simulink library "can_control"  (R2023b)
settings: Solver=VariableStepAuto  StartTime=0.0  StopTime=10.0  RelTol=1e-3
undefined symbols (not defined in the file or in its folder): Data, Error, Extended, ID, Length, Remote, Timestamp
libraries: simulink x3, $bdroot x2, dspswit3 x1
settings Model: Creator=Olga  LastModifiedBy=Olga
settings SFSimCC: SimCustomHeaderCode="#include \"can_control.h\""  SimUserSources=.\can_control.c  SimAnalyzeCustomCode=on
settings RTWCC: RTWUseSimCustomCode=on  CustomHeaderCode="#include \"can_control.h\""  CustomSource=.\can_control.c

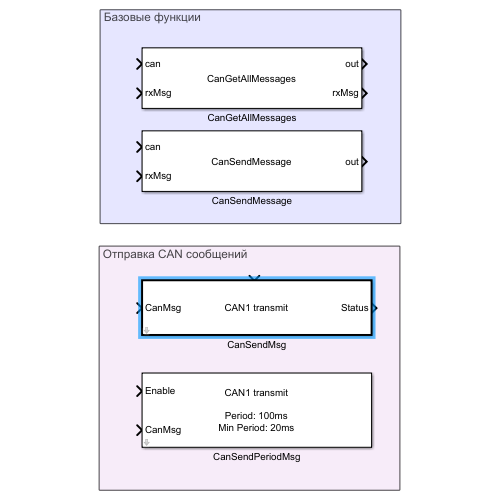
[thumbnail: Simulink's stored preview of the top-level diagram]
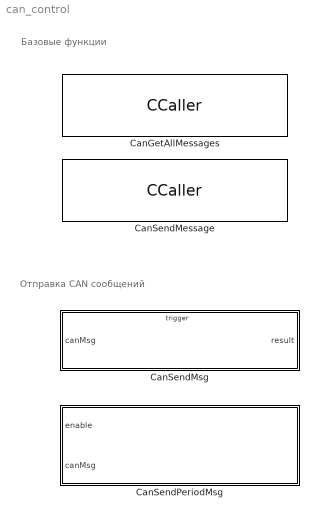
== system can_control ==
  note: Базовые функции
  note: Отправка CAN сообщений
  CanGetAllMessages : CCaller  FunctionName=CanGetAllMessages  PortSpecificationStruct="%)30     .    > 4   8    (     @         %    \"     ,    !     0         %  0 \"0    $    _    07)G3F%M90  4&]R=$YA;64 4V-O<&4     26YD97@     5'EP90      4VEZ90      27-';&]B86P   X    P    !@    @    $          4    (     0    ,    !         !   P!O=70 #@   #     &    \"     0         !0    @    !     P    $         $  # &]U=  .    .     8    (    !          %    \"     $    &     0         0    !@   $]U='!U=   #@   #@    &    \"     8         !0    @    !     0    $         \"0    @               X    X    !@    @    $          4    (     0    <    !         !     '    8F]O;&5A;@ .    ,     8    (    !          %    \"     $    !     0         0  $ ,0    X    P    !@    @    ) @        4    (     0    $    !          (  0      #@   #     &    \"     0         !0    @    !     P    $         $  # &-A;@ .    ,     8    (    !          %    \"     $    #     0         0  , 8V%N  X    X    !@    @    $          4    (     0    4    !         !     %    26YP=70    .    .     8    (    !@         %    \"     $    !     0         )    \"               #@   #@    &    \"     0         !0    @    !    !0    $         $     4   !I;G0S,@    X    P    !@    @    $          4    (     0    $    !         !   0 Q    #@   #     &    \"     D\"        !0    @    !     0    $          @ !       .    .     8    (    !          %    \"     $    %     0         0    !0   ')X37-G    #@   #@    &    \"     0         !0    @    !    !0    $         $     4   !R>$US9P    X   !     !@    @    $          4    (     0    L    !         !     +    26YP=71/=71P=70       X    X    !@    @    &          4    (     0    $    !          D    (            \\#\\.    0     8    (    !          %    \"     $    .     0         0    #@   $)U<SH@0T%.7TUS9U]T   .    ,     8    (    !          %    \"     $    \"     0         0  ( +3$   X    P    !@    @    ) @        4    (     0    $    !          (  0"
  CanSendMessage : CCaller  FunctionName=CanSendMessage  PortSpecificationStruct="%)30     .    < 4   8    (     @         %    \"     ,    !     0         %  0 \"0    $    _    07)G3F%M90  4&]R=$YA;64 4V-O<&4     26YD97@     5'EP90      4VEZ90      27-';&]B86P   X    P    !@    @    $          4    (     0    ,    !         !   P!O=70 #@   #     &    \"     0         !0    @    !     P    $         $  # &]U=  .    .     8    (    !          %    \"     $    &     0         0    !@   $]U='!U=   #@   #@    &    \"     8         !0    @    !     0    $         \"0    @               X    X    !@    @    $          4    (     0    <    !         !     '    8F]O;&5A;@ .    ,     8    (    !          %    \"     $    !     0         0  $ ,0    X    P    !@    @    ) @        4    (     0    $    !          (  0      #@   #     &    \"     0         !0    @    !     P    $         $  # &-A;@ .    ,     8    (    !          %    \"     $    #     0         0  , 8V%N  X    X    !@    @    $          4    (     0    4    !         !     %    26YP=70    .    .     8    (    !@         %    \"     $    !     0         )    \"               #@   #@    &    \"     0         !0    @    !    !0    $         $     4   !I;G0S,@    X    P    !@    @    $          4    (     0    $    !         !   0 Q    #@   #     &    \"     D\"        !0    @    !     0    $          @ !       .    .     8    (    !          %    \"     $    %     0         0    !0   ')X37-G    #@   #@    &    \"     0         !0    @    !    !0    $         $     4   !R>$US9P    X    X    !@    @    $          4    (     0    4    !         !     %    26YP=70    .    .     8    (    !@         %    \"     $    !     0         )    \"            / _#@   $     &    \"     0         !0    @    !    #@    $         $     X   !\"=7,Z($-!3E]-<V=?=   #@   #     &    \"     0         !0    @    !     @    $         $  \" \"TQ   .    ,     8    (    \"0(        %    \"     $    !     0         \"  $"
  СanSendMsg : Subsystem  mask(Отправка сообщения CAN){can=CAN1}
      mask help:
      | Выберите CAN шину для передачи сообщения.
      |
      | Порт canMsg - Сообщение для отправки типа Bus: CAN_MESSAGE_BUS.
      |
      | Данный блок, при вызове, поместит сообщений в очередь CAN для отправки.
      |
      | Status - статус выполнения функции boolean
      mask init:
      | blockName = "CAN" + num2str(can) + " transmit";
      mask TypeOptions can: CAN1 | CAN2
      mask DialogControl ParameterGroupVar Prompt: Параметры
      mask Display:
      | disp(blockName);
      | port_label('input', 1, 'CanMsg');
      | port_label('output', 1, 'Status');
  СanSendPeriodMsg : Subsystem  mask(CanSend){by_period=on, by_dataChange=off, can=CAN1, period_time=0.1, sample_time=0.02}
      mask prompts: by_period "Периодическая отправка"; by_dataChange "По изменению данных"; period_time "Период , сек:"; sample_time "Минимальный период, сек:"
      mask help: Выберите CAN шину для передачи сообщения.<br>Sample time - период выполнения блока. Должен быть больше шага моделирования. Значение -1 задаёт Sample time как наследуемый.<br><br>-Порт enable - включения/выключения отправки.<br>-Порт canMsg - Сообщение для отправки типа Bus: CAN_MESSAGE_BUS(можно создать коммандой canMessageBusType, скопировать и поместить в словарь модели)
      mask init:
      | block_name = "CAN" + num2str(can) + " transmit";
      | period = num2str(period_time * 1000)+ "ms";
      | 
      | if(sample_time == -1)
      |     min_period = "Inherit";
      | else
      |     min_period = num2str(sample_time * 1000)+ "ms";  
      | end
      | 
      | if(by_period == true && by_dataChange == false)
      |     block_name = "CAN" + num2str(can) + " transmit\n\n" + "Period: " + period + "\nMin Period: " + min_period;
      | elseif(by_period == true && by_dataChange == true)
      |     block_name = "CAN" + num2str(can) + " transmit\n\n" + "By Data Change\n" + "Period: " + period + "\nMin Period: " + min_period;
      | elseif(by_period == false && by_dataChange == true)
      |     block_name = "CAN" + num2str(can) + " transmit\n\n" + "By Data Change" + "\nMin Period: " + min_period;
      | else
      |     block_name = "CAN" + num2str(can) + " transmit OFF";
      | end
      mask TypeOptions can: CAN1 | CAN2
      mask DialogControl Container4 Prompt: Настройки:
      mask DialogControl ParameterGroupVar Prompt: Параметры
      mask DialogControl Container3 Prompt: Периоды
      mask Display:
      | disp(block_name);
      | port_label('input', 1, 'Enable');
      | port_label('input', 2, 'CanMsg');

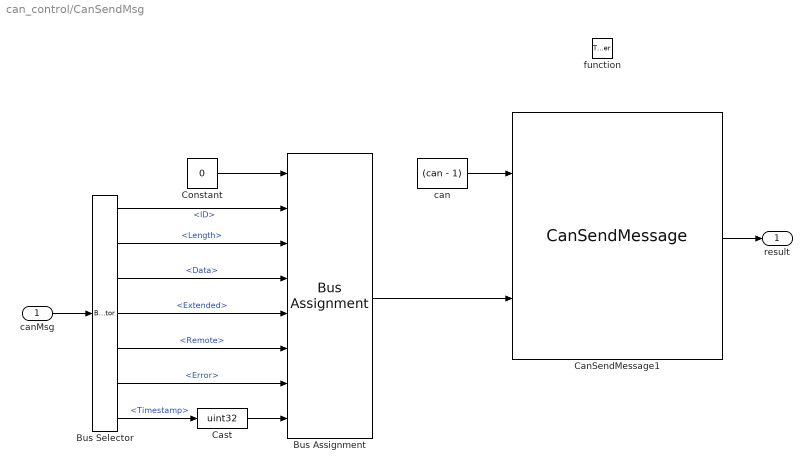
== system can_control/СanSendMsg ==
  canMsg : Inport  OutDataTypeStr=Bus: CAN_MESSAGE_BUS
  function : TriggerPort  TriggerType=function-call  VariantControl=(inherit)
  Bus Assignment : BusAssignment  AssignedSignals=ID,Length,Data,Extended,Remote,Error,Timestamp
  Bus Selector : BusSelector  OutputSignals=ID,Length,Data,Extended,Remote,Error,Timestamp
  CanSendMessage1 : $bdroot/CanSendMessage  SampleTime=-1
  Cast : DataTypeConversion  OutDataTypeStr=uint32  RndMeth=Simplest  SaturateOnIntegerOverflow=off
  Constant : Constant  Value=0  OutDataTypeStr=Bus: CAN_Msg_t
  can : Constant  Value=(can - 1)  OutDataTypeStr=int32
  result : Outport  OutDataTypeStr=boolean
  wires:
  canMsg/1 -> Bus Selector/1
  can/1 -> CanSendMessage1/1
  Bus Assignment/1 -> CanSendMessage1/2
  Constant/1 -> Bus Assignment/1
  Bus Selector/1 -> Bus Assignment/2  "<ID>"
  Bus Selector/2 -> Bus Assignment/3  "<Length>"
  Bus Selector/3 -> Bus Assignment/4  "<Data>"
  Bus Selector/4 -> Bus Assignment/5  "<Extended>"
  Bus Selector/5 -> Bus Assignment/6  "<Remote>"
  Bus Selector/6 -> Bus Assignment/7  "<Error>"
  Bus Selector/7 -> Cast/1  "<Timestamp>"
  CanSendMessage1/1 -> result/1
  Cast/1 -> Bus Assignment/8

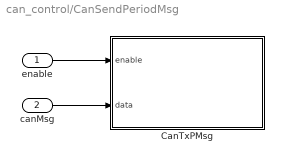
== system can_control/СanSendPeriodMsg ==
  enable : Inport  OutDataTypeStr=boolean
  canMsg : Inport  Port=2  OutDataTypeStr=Bus: CAN_MESSAGE_BUS
  CanTxPMsg : Subsystem  TreatAsAtomicUnit=on  SystemSampleTime=sample_time
  wires:
  canMsg/1 -> CanTxPMsg/2(data)
  enable/1 -> CanTxPMsg/1(enable)

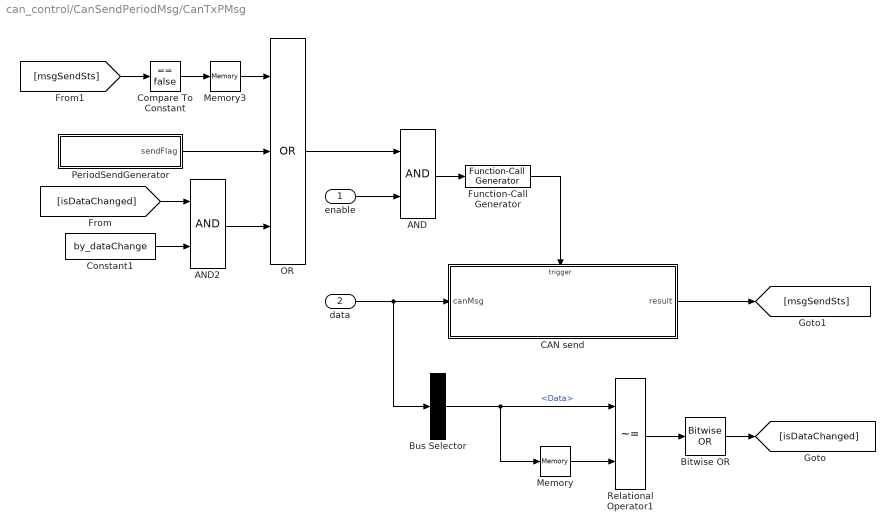
== system can_control/СanSendPeriodMsg/CanTxPMsg ==
  enable : Inport  OutDataTypeStr=boolean
  data : Inport  Port=2
  AND : Logic  AllPortsSameDT=off  OutDataTypeStr=boolean
  AND2 : Logic  AllPortsSameDT=off  OutDataTypeStr=boolean
  Bitwise OR : simulink/Logic and Bit Operations/Bitwise Operator  logicop=OR  UseBitMask=off  BitMask=bin2dec('11011001')  BitMaskRealWorld=Stored Integer
      settings: LibrarySourceBlock=|
      | simulink/Quick Insert/Logic and Bit
      | Operations/Bitwise OR
  Bus Selector : BusSelector  OutputSignals=Data
  CAN send : Subsystem  TreatAsAtomicUnit=on
  Compare To Constant : simulink/Logic and Bit Operations/Compare To Constant  relop===  const=false  OutDataTypeStr=boolean  ZeroCross=off
  Constant1 : Constant  Value=by_dataChange  OutDataTypeStr=boolean
  Function-Call Generator : simulink/Ports & Subsystems/Function-Call Generator  sample_time=sample_time  numberOfIterations=1  DisallowWideOutput=off  ShowEnablePort=on
  Memory : Memory  InheritSampleTime=on
  Memory3 : Memory  InheritSampleTime=on
  OR : Logic  Operator=OR  Inputs=3  AllPortsSameDT=off  OutDataTypeStr=boolean
  PeriodSendGenerator : Subsystem
  Relational Operator1 : RelationalOperator  Operator=~=  OutDataTypeStr=boolean  RndMeth=Simplest  InputSameDT=off
  wires:
  PeriodSendGenerator/1(sendFlag) -> OR/2
  [msgSendSts] -> Compare To Constant/1
  CAN send/1(result) -> [msgSendSts]
  Compare To Constant/1 -> Memory3/1
  [isDataChanged] -> AND2/1
  enable/1 -> AND/2
  AND/1 -> Function-Call Generator/1
  Bitwise OR/1 -> [isDataChanged]
  Constant1/1 -> AND2/2
  Function-Call Generator/1 -> CAN send/Trigger
  Memory/1 -> Relational Operator1/2
  AND2/1 -> OR/3
  Relational Operator1/1 -> Bitwise OR/1
  Bus Selector/1 -> Relational Operator1/1, Memory/1  "<Data>"
  data/1 -> Bus Selector/1, CAN send/1(canMsg)
  Memory3/1 -> OR/1
  OR/1 -> AND/1

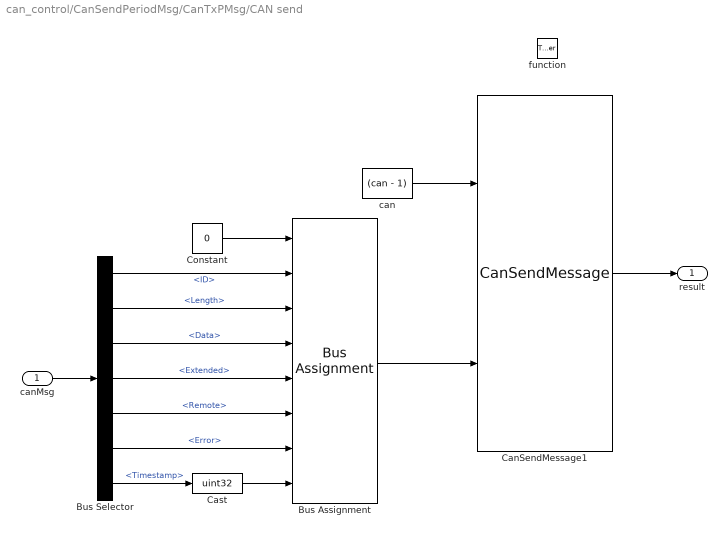
== system can_control/СanSendPeriodMsg/CanTxPMsg/CAN send ==
  canMsg : Inport  OutDataTypeStr=Bus: CAN_MESSAGE_BUS
  function : TriggerPort  TriggerType=function-call  VariantControl=(inherit)
  Bus Assignment : BusAssignment  AssignedSignals=ID,Length,Data,Extended,Remote,Error,Timestamp
  Bus Selector : BusSelector  OutputSignals=ID,Length,Data,Extended,Remote,Error,Timestamp
  CanSendMessage1 : $bdroot/CanSendMessage  SampleTime=-1
  Cast : DataTypeConversion  OutDataTypeStr=uint32  RndMeth=Simplest  SaturateOnIntegerOverflow=off
  Constant : Constant  Value=0  OutDataTypeStr=Bus: CAN_Msg_t
  can : Constant  Value=(can - 1)  OutDataTypeStr=int32
  result : Outport  OutDataTypeStr=boolean
  wires:
  CanSendMessage1/1 -> result/1
  can/1 -> CanSendMessage1/1
  Bus Selector/7 -> Cast/1  "<Timestamp>"
  Bus Selector/3 -> Bus Assignment/4  "<Data>"
  Bus Selector/2 -> Bus Assignment/3  "<Length>"
  Bus Selector/1 -> Bus Assignment/2  "<ID>"
  Bus Selector/6 -> Bus Assignment/7  "<Error>"
  Constant/1 -> Bus Assignment/1
  Bus Selector/5 -> Bus Assignment/6  "<Remote>"
  Bus Assignment/1 -> CanSendMessage1/2
  Bus Selector/4 -> Bus Assignment/5  "<Extended>"
  canMsg/1 -> Bus Selector/1
  Cast/1 -> Bus Assignment/8

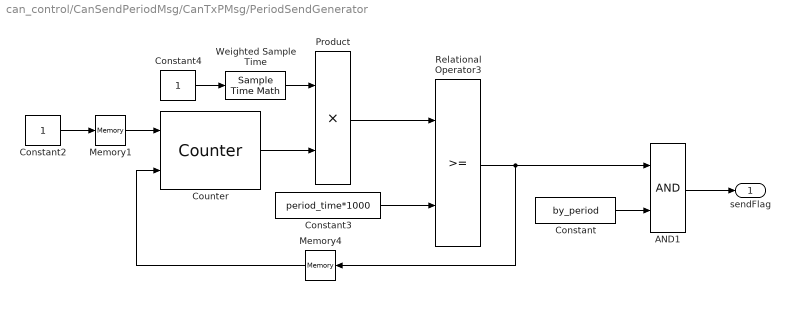
== system can_control/СanSendPeriodMsg/CanTxPMsg/PeriodSendGenerator ==
  AND1 : Logic  AllPortsSameDT=off  OutDataTypeStr=boolean
  Constant : Constant  Value=by_period  OutDataTypeStr=boolean
  Constant2 : Constant  OutDataTypeStr=uint32
  Constant3 : Constant  Value=period_time*1000  OutDataTypeStr=uint32
  Constant4 : Constant  OutDataTypeStr=uint32
  Counter : dspswit3/Counter  Direction=Up  CountEvent=Non-zero sample  CounterSize=32 bits  MaxCount=255  InitialCount=0  Output=Count  HitValue=32  ResetInput=on  SamplesPerFrame=1  Ts=-1  CntDtype=uint32  HitDtype=Logical
  Memory1 : Memory  InheritSampleTime=on
  Memory4 : Memory  InheritSampleTime=on
  Product : Product  OutDataTypeStr=uint32  RndMeth=Simplest
  Relational Operator3 : RelationalOperator  OutDataTypeStr=boolean  ZeroCross=off  RndMeth=Simplest  InputSameDT=off
  Weighted Sample Time : SampleTimeMath  TsampMathOp=Ts Only  weightValue=uint32(1000)  OutDataTypeStr=single
  sendFlag : Outport
  wires:
  Constant3/1 -> Relational Operator3/2
  Relational Operator3/1 -> Memory4/1, AND1/1
  Memory1/1 -> Counter/1
  Constant4/1 -> Weighted Sample Time/1
  AND1/1 -> sendFlag/1
  Memory4/1 -> Counter/2
  Constant2/1 -> Memory1/1
  Weighted Sample Time/1 -> Product/1
  Constant/1 -> AND1/2
  Product/1 -> Relational Operator3/1
  Counter/1 -> Product/2
